simulink model "model_2015aQPSK1"  (R2015a)
settings: Solver=FixedStepDiscrete  SolverMode=SingleTasking  StartTime=0.0  StopTime=inf  RelTol=1e-3
libraries: commutil2 x2, commfilt2 x2, dspsrcs4 x2, commchan3 x1, commsink2 x1, commrandsrc2 x1, dspsigops x1
settings Model: Creator=com_1  LastModifiedBy=igiliev

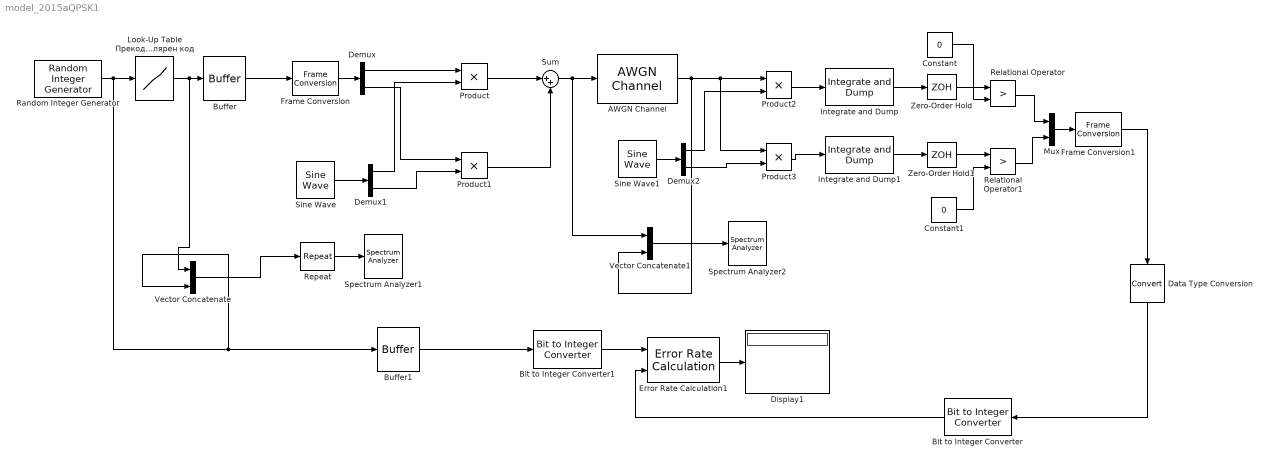
== system model_2015aQPSK1 ==
  AWGN Channel : commchan3/AWGN Channel  InputProcessing=Columns as channels (frame based)  seed=12397  noiseMode="Signal to noise ratio  (Eb/No)"  EbNodB=6  EsNodB=10  SNRdB=10  bitsPerSym=1  Ps=1  Tsym=2  variance=1
  Bit to Integer Converter : commutil2/Bit to Integer Converter  nbits=2  bitOrder=MSB first  signedOutputValues=Unsigned  outDtype=Inherit via internal rule  outDtypeSigned=Inherit via internal rule
  Bit to Integer Converter1 : commutil2/Bit to Integer Converter  nbits=2  bitOrder=MSB first  signedOutputValues=Unsigned  outDtype=Inherit via internal rule  outDtypeSigned=Inherit via internal rule
  Buffer : Buffer  N=2  TreatMby1Signals=One channel
  Buffer1 : Buffer  N=2  TreatMby1Signals=One channel
  Constant : Constant  Value=0
  Constant1 : Constant  Value=0
  Data Type Conversion : DataTypeConversion
  Demux : Demux  Outputs=2
  Demux1 : Demux  Outputs=2
  Demux2 : Demux  Outputs=2
  Display1 : Display
  Error Rate Calculation1 : commsink2/Error Rate Calculation  N=1  st_delay=1  cp_mode=Entire frame  subframe=[]  PMode=Port  WsName=ErrorVec  RsMode2=off  stop=off  numErr=100  maxBits=1e6
  Frame Conversion : FrameConversion  OutFrame=Sample-based
  Frame Conversion1 : FrameConversion
  Integrate and Dump : commfilt2/Integrate and Dump  obssamples=100  offsetsamples=0  nodump=off  roundingMode=Floor  overflowMode=off
  Integrate and Dump1 : commfilt2/Integrate and Dump  obssamples=100  offsetsamples=0  nodump=off  roundingMode=Floor  overflowMode=off
  Look-Up Table Прекодер в биполярен код : Lookup  InputValues=[0 1]  Table=[-1 1]  SaturateOnIntegerOverflow=on
  Mux : Mux  Inputs=2
  Product{,1..3} (4 alike) : Product
  Random Integer Generator : commrandsrc2/Random Integer Generator  mul=2  seed=37  Ts=1  frameBased=off  sampPerFrame=1  orient=off  outDataType=double
  Relational Operator : RelationalOperator  Operator=>  OutDataTypeStr=boolean
  Relational Operator1 : RelationalOperator  Operator=>  OutDataTypeStr=boolean
  Repeat : dspsigops/Repeat  N=10  RateOptions=Allow multirate processing  ic=0  mode=Unused parameter value
  Sine Wave : dspsrcs4/Sine Wave  Amplitude=[1 -1]  Frequency=5  Phase=[0 pi/2]  SampleMode=Discrete  OutComplex=Real  CompMethod=Trigonometric fcn  TableSize=Speed  SampleTime=1/50  SamplesPerFrame=1  ResetState=Restart at time zero  dataType=double  wordLen=16  udDataType=sfix(16)  fracBitsMode=Best precision  numFracBits=15  OutDataTypeStr=double  LastOutDataTypeStr=double
  Sine Wave1 : dspsrcs4/Sine Wave  Amplitude=[1 -1]  Frequency=5  Phase=[0 pi/2]  SampleMode=Discrete  OutComplex=Real  CompMethod=Trigonometric fcn  TableSize=Speed  SampleTime=1/50  SamplesPerFrame=1  ResetState=Restart at time zero  dataType=double  wordLen=16  udDataType=sfix(16)  fracBitsMode=Best precision  numFracBits=15  OutDataTypeStr=double  LastOutDataTypeStr=double
  Spectrum Analyzer1 : SpectrumAnalyzer
  Spectrum Analyzer2 : SpectrumAnalyzer
  Sum : Sum  Inputs=|++
  Vector Concatenate : Concatenate  Mode=Multidimensional array  ConcatenateDimension=2
  Vector Concatenate1 : Concatenate  Mode=Multidimensional array  ConcatenateDimension=2
  Zero-Order Hold : ZeroOrderHold  SampleTime=2
  Zero-Order Hold1 : ZeroOrderHold  SampleTime=2
  wires:
  Random Integer Generator/1 -> Vector Concatenate/2, Buffer1/1, Look-Up Table Прекодер в биполярен код/1
  Frame Conversion/1 -> Demux/1
  Product/1 -> Sum/1
  Sine Wave/1 -> Demux1/1
  Product1/1 -> Sum/2
  Demux1/2 -> Product1/2
  Demux1/1 -> Product/2
  Demux/1 -> Product/1
  Demux/2 -> Product1/1
  Sum/1 -> Vector Concatenate1/1, AWGN Channel/1
  AWGN Channel/1 -> Vector Concatenate1/2, Product3/1, Product2/1
  Product2/1 -> Integrate and Dump/1
  Product3/1 -> Integrate and Dump1/1
  Integrate and Dump/1 -> Zero-Order Hold/1
  Integrate and Dump1/1 -> Zero-Order Hold1/1
  Zero-Order Hold1/1 -> Relational Operator1/1
  Constant1/1 -> Relational Operator1/2
  Zero-Order Hold/1 -> Relational Operator/1
  Constant/1 -> Relational Operator/2
  Relational Operator/1 -> Mux/1
  Relational Operator1/1 -> Mux/2
  Mux/1 -> Frame Conversion1/1
  Error Rate Calculation1/1 -> Display1/1
  Frame Conversion1/1 -> Data Type Conversion/1
  Buffer1/1 -> Bit to Integer Converter1/1
  Buffer/1 -> Frame Conversion/1
  Sine Wave1/1 -> Demux2/1
  Demux2/1 -> Product2/2
  Demux2/2 -> Product3/2
  Repeat/1 -> Spectrum Analyzer1/1
  Look-Up Table Прекодер в биполярен код/1 -> Vector Concatenate/1, Buffer/1
  Vector Concatenate/1 -> Repeat/1
  Data Type Conversion/1 -> Bit to Integer Converter/1
  Bit to Integer Converter/1 -> Error Rate Calculation1/2
  Bit to Integer Converter1/1 -> Error Rate Calculation1/1
  Vector Concatenate1/1 -> Spectrum Analyzer2/1
